simulink model "Speed_control_with_reduced_model_order"  (R2016b)
settings: Solver=ode45  StartTime=0.0  StopTime=1  FixedStep=0.0000001  RelTol=1e-4
settings Model: Creator=emilio  LastModifiedBy=danielesmn

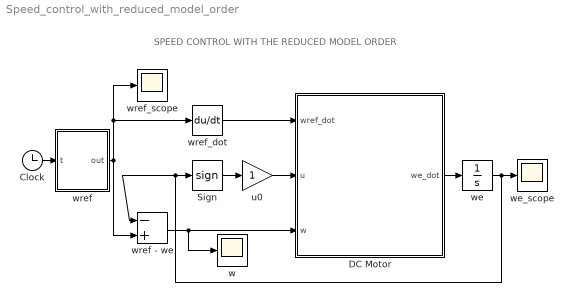
== system Speed_control_with_reduced_model_order ==
  note: SPEED CONTROL WITH THE REDUCED MODEL ORDER
  Clock : Clock
  DC Motor : MATLAB Function  TreatAsAtomicUnit=on
  Sign : Signum  ZeroCross=off
  u0 : Gain
  w : Scope
  we : Integrator
  we_scope : Scope
  wref : MATLAB Function  TreatAsAtomicUnit=on
  wref - we : Sum  Inputs=-+
  wref_dot : Derivative
  wref_scope : Scope
  wires:
  DC Motor/1(we_dot) -> we/1
  we/1 -> we_scope/1, Sign/1, wref - we/1
  wref_dot/1 -> DC Motor/1(wref_dot)
  wref - we/1 -> w/1, DC Motor/3(w)
  Sign/1 -> u0/1
  u0/1 -> DC Motor/2(u)
  Clock/1 -> wref/1(t)
  wref/1(out) -> wref - we/2, wref_scope/1, wref_dot/1

== matlab function Speed_control_with_reduced_model_order/DC Motor ==
  data: wref_dot input; u input; we_dot output; w input
function we_dot = DC_Motor(wref_dot, u, w)

%Reduced model of the DC Motor

R = 0.5;          %Armature resistance (Ohm)
kt = 0.008;       %Torque constant (Nm/A)
J = 0.001;        %Inertia of the motor rotor (Kg*m^2)
B = 0.01;         %Coefficient of viscous friction (Nm*s/rad)
lambda0 = 0.001;  %Back electromotive force (EMF) constant (V*s/rad)


we_dot = kt*lambda0/(J*R)*w - kt/(J*R)*u + B/J*w + wref_dot;

== matlab function Speed_control_with_reduced_model_order/wref ==
  data: t input; out output
function out = input(t)

if t < 0.5
    out = 1;
else
    out = -1;
end
